simulink model "vehicleDynamics"  (R2016b)
settings: Solver=FixedStepAuto  StartTime=0.0  StopTime=10.0  RelTol=1e-3  EnableMultiTasking=on
settings Model: Creator=Josef  LastModifiedBy=NEATdemo
settings OptimizationCC: LifeSpan=inf
settings DebuggingCC: SFUnexpectedBacktrackingDiag=warning  SFNoUnconditionalDefaultTransitionDiag=warning  SFExecutionAtInitializationDiag=none
settings GRTTargetCC: TargetLangStandard=C89/C90 (ANSI)
settings ConfigComp: CovMetricSettings=dw  CovHtmlReporting=on  CovSaveCumulativeToWorkspaceVar=on  CovSaveSingleToWorkspaceVar=on  CovExternalEMLEnable=off

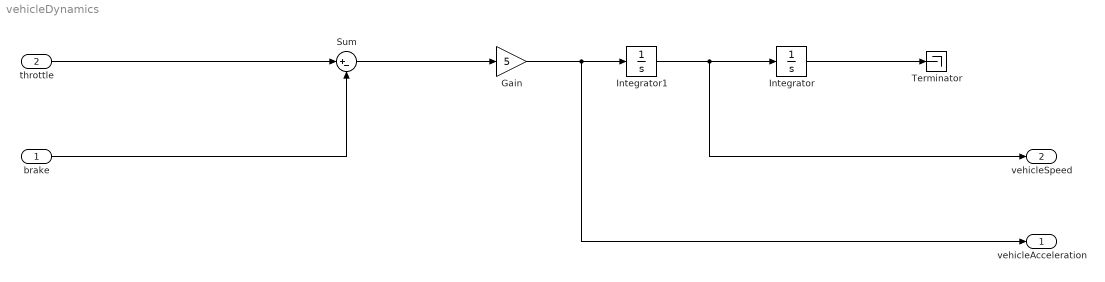
== system vehicleDynamics ==
  brake : Inport
      settings: AttributesFormatString=driverBrake
  throttle : Inport  Port=2
      settings: AttributesFormatString=driverThrottle
  Gain : Gain  Gain=5
  Integrator : Integrator
  Integrator1 : Integrator  LimitOutput=on  LowerSaturationLimit=0
  Sum : Sum  Inputs=|+-
  Terminator : Terminator
  vehicleAcceleration : Outport
      settings: AttributesFormatString=acceleration
  vehicleSpeed : Outport  Port=2
      settings: AttributesFormatString=speed
  wires:
  Integrator1/1 -> vehicleSpeed/1, Integrator/1
  Sum/1 -> Gain/1
  Gain/1 -> vehicleAcceleration/1, Integrator1/1
  Integrator/1 -> Terminator/1
  throttle/1 -> Sum/1
  brake/1 -> Sum/2
